simulink model "multirotor_simulation"  (R2025b)
settings: Solver=ode4  StartTime=0.0  StopTime=21  FixedStep=ST  RelTol=1e-3
values from neighbouring files (symbols this model uses):
  a0 = 0    [multirotor_start.m]
  ASLOPE = 5.9    [multirotor_start.m]
  Ax = 0.023    [multirotor_start.m]
  Ay = 0.023    [multirotor_start.m]
  Az = 0.106    [multirotor_start.m]
  BLADES = 2    [multirotor_start.m]
  BLCG = 0    [multirotor_start.m]
  BLCP = 0    [multirotor_start.m]
  BLH1 = b*sind(30)    [multirotor_start.m]
  BLH2 = b    (= 0.275)    [multirotor_start.m]
  BLH3 = b*sind(30)    [multirotor_start.m]
  BLH4 = -b*sind(30)    [multirotor_start.m]
  BLH5 = -b    (= -0.275)    [multirotor_start.m]
  BLH6 = -b*sind(30)    [multirotor_start.m]
  chi1 = 1    [multirotor_start.m]
  chi2 = -1    [multirotor_start.m]
  chi3 = 1    [multirotor_start.m]
  chi4 = -1    [multirotor_start.m]
  chi5 = 1    [multirotor_start.m]
  chi6 = -1    [multirotor_start.m]
  CHORD = 17.55e-3    (= 0.01755)    [multirotor_start.m]
  CHORD75 = 21e-3    (= 0.021)    [multirotor_start.m]
  controller_mode = 1    [multirotor_start.m]
  del_sp = [0 0.7 0 0]'    [multirotor_start.m]
  dyn_visco = 17.89e-6    (= 1.789e-05)    [multirotor_start.m]
  g0 = 9.80665    [multirotor_start.m]
  href = 0    [multirotor_start.m]
  k_ind = 1.35    [multirotor_start.m]
  k_Omega = 14.92    [multirotor_start.m]
  latref = 44.200626    [multirotor_start.m]
  lonref = 12.063822    [multirotor_start.m]
  m = 2.15    [multirotor_start.m]
  MC_ATT_PITCH = 30*pi/180    (= 0.523598775598)    [multirotor_start.m]
  MC_ATT_ROLL = 30*pi/180    (= 0.523598775598)    [multirotor_start.m]
  MC_ATT_YAW = 180*pi/180    (= 3.14159265359)    [multirotor_start.m]
  MC_PITCH_P = 3    [multirotor_start.m]
  MC_PITCHRATE_D = 0    [multirotor_start.m]
  MC_PITCHRATE_I = 0.1*0.5    (= 0.05)    [multirotor_start.m]
  MC_PITCHRATE_P = 0.09    [multirotor_start.m]
  MC_ROLL_P = 3    [multirotor_start.m]
  MC_ROLLRATE_D = 0    [multirotor_start.m]
  MC_ROLLRATE_I = 0.1*0.5    (= 0.05)    [multirotor_start.m]
  MC_ROLLRATE_P = 0.09    [multirotor_start.m]
  MC_VEL_FWD = 5    [multirotor_start.m]
  MC_VEL_FWD_OPT = 0.5    [multirotor_start.m]
  MC_VEL_LAT = 5    [multirotor_start.m]
  MC_VEL_LAT_OPT = 0.5    [multirotor_start.m]
  MC_VEL_VERT = 1    [multirotor_start.m]
  MC_YAW_P = 1.8*0.5    (= 0.9)    [multirotor_start.m]
  MC_YAWRATE_D = 0    [multirotor_start.m]
  MC_YAWRATE_I = 0.1*0    (= 0)    [multirotor_start.m]
  MC_YAWRATE_P = 0.175*0.4    (= 0.07)    [multirotor_start.m]
  MPC_XY_VEL_D_ACC = 0.2*2    (= 0.4)    [multirotor_start.m]
  MPC_XY_VEL_I_ACC = 0.8    [multirotor_start.m]
  MPC_XY_VEL_P_ACC = 1.7*3/3    (= 1.7)    [multirotor_start.m]
  MPC_Z_VEL_D_ACC = 0    [multirotor_start.m]
  MPC_Z_VEL_I_ACC = 2    [multirotor_start.m]
  MPC_Z_VEL_P_ACC = 4    [multirotor_start.m]
  n = 0.6359    [multirotor_start.m]
  p00 = 7.145e-2    (= 0.07145)    [multirotor_start.m]
  p01 = 0.4377    [multirotor_start.m]
  p02 = -10.13    [multirotor_start.m]
  p10 = 1.259e-3    (= 0.001259)    [multirotor_start.m]
  p11 = 1.284e-3    (= 0.001284)    [multirotor_start.m]
  p20 = -7.513e-7    (= -7.513e-07)    [multirotor_start.m]
  PWM_hover = (PWM_idle+PWM_max)/2    (= 1550)    [multirotor_start.m]
  PWM_idle = 1100    [multirotor_start.m]
  PWM_max = 2000    [multirotor_start.m]
  ROTOR = 4*0.0254    (= 0.1016)    [multirotor_start.m]
  set_point_input = 0    [multirotor_start.m]
  ST = 0.01    [multirotor_start.m]
  STACG = 0    [multirotor_start.m]
  STACP = 0    [multirotor_start.m]
  STAH1 = -b*cosd(30)    [multirotor_start.m]
  STAH2 = 0    [multirotor_start.m]
  STAH3 = b*cosd(30)    [multirotor_start.m]
  STAH4 = b*cosd(30)    [multirotor_start.m]
  STAH5 = 0    [multirotor_start.m]
  STAH6 = -b*cosd(30)    [multirotor_start.m]
  TERMINAL_SPEED = 0.5    [multirotor_start.m]
  Theta0 = 45*pi/180    (= 0.785398163397)    [multirotor_start.m]
  THETT = -38.0973*pi/180    (= -0.66492332112)    [multirotor_start.m]
  V_sin_x = 0.3    [multirotor_start.m]
  Vsp = [0 1 0]'    [multirotor_start.m]
  wind_rate = [0 0 0]'    [multirotor_start.m]
  wind_velocity_e = [0 0 0]'    [multirotor_start.m]
  WLCG = -0.03    [multirotor_start.m]
  WLCP = -0.08    [multirotor_start.m]
  WLH1 = 32e-3    (= 0.032)    [multirotor_start.m]
  WLH2 = 32e-3    (= 0.032)    [multirotor_start.m]
  WLH3 = 32e-3    (= 0.032)    [multirotor_start.m]
  WLH4 = 32e-3    (= 0.032)    [multirotor_start.m]
  WLH5 = 32e-3    (= 0.032)    [multirotor_start.m]
  WLH6 = 32e-3    (= 0.032)    [multirotor_start.m]
  Xe_target = Xe_0 + [2, 3, -10]'    [multirotor_start.m]
undefined symbols (not defined in the file or in its folder): fspecial, gray, Rec, SDTV, Sim3dSensor, X, Y, Z
libraries: sm_lib x258, slpidlib x18, nesl_utility x15, sharedtransform x4, simulink x3, aerolibanimutils x2, sim3dcameralib x2, dspvision x2, uavsim3dlib x2, aerolibutil x2, visionconversions x1, visionanalysis x1
(part 1 of 10)
settings Model: Creator=pries  LastModifiedBy=pries
settings RTWCC: GPUComputeCapability=3.5

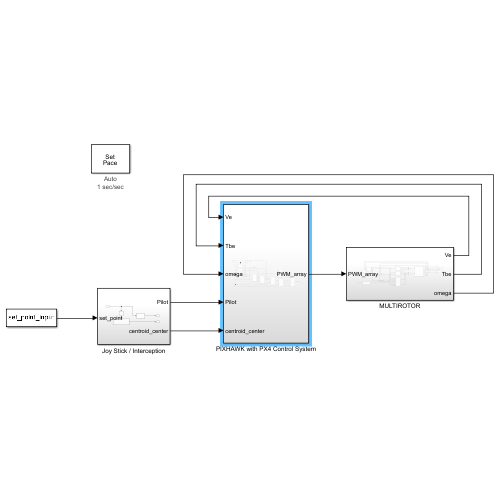
[thumbnail: Simulink's stored preview of the top-level diagram]
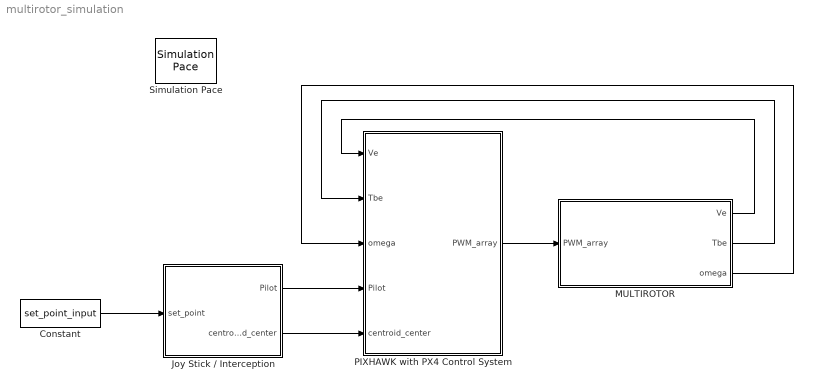
== system multirotor_simulation ==
  Constant : Constant  Value=set_point_input
  Joy Stick / Interception : Subsystem
  MULTIROTOR : Subsystem
  PIXHAWK with PX4 Control System : Subsystem
  Simulation Pace : aerolibanimutils/Simulation Pace  SimulationPace=1  SleepMode=Auto  OutputPaceError=off  SampleTime=ST
  wires:
  PIXHAWK with PX4 Control System/1(PWM_array) -> MULTIROTOR/1(PWM_array)
  MULTIROTOR/1(Ve) -> PIXHAWK with PX4 Control System/1(Ve)
  MULTIROTOR/2(Tbe) -> PIXHAWK with PX4 Control System/2(Tbe)
  MULTIROTOR/3(omega) -> PIXHAWK with PX4 Control System/3(omega)
  Constant/1 -> Joy Stick / Interception/1(set_point)
  Joy Stick / Interception/1(Pilot) -> PIXHAWK with PX4 Control System/4(Pilot)
  Joy Stick / Interception/2(centroid_center) -> PIXHAWK with PX4 Control System/5(centroid_center)

== system multirotor_simulation/Joy Stick // Interception ==
  set_point : Inport
  Compare To Constant : simulink/Logic and Bit Operations/Compare To Constant  relop===  const=0  OutDataTypeStr=boolean
  GCS : Subsystem
  HUSKYLENS : Subsystem
  Pilot : Outport
  centroid_center : Outport  Port=2
  wires:
  HUSKYLENS/1(centroid_center) -> centroid_center/1
  Compare To Constant/1 -> HUSKYLENS/Enable
  GCS/1(Pilot) -> Pilot/1
  set_point/1 -> Compare To Constant/1, GCS/1(set_point)

== system multirotor_simulation/MULTIROTOR ==
  PWM_array : Inport
  3D : Subsystem
  6DOF (Euler Angles) : aerolibobsolete/6DOF (Euler Angles)  units=Metric (MKS)  mtype=Fixed  rep=Euler Angles  xme_0=Xe_0  Vm_0=V0  eul_0=euler0  pm_0=omega0  mass_0=m  mass_e=0.5  mass_f=2.0  inertia=J  inertia_e=eye(3)  inertia_f=2*eye(3)  k_quat=1.0  vre_flag=on  abi_flag=off  aMode=0  xme_statename=''  Vm_statename=''  eul_statename=''  quat_statename=''  pm_statename=''  mass_statename=''
  Add : Sum  Inputs=+++
  Add1 : Sum  Inputs=+++
  Add2 : Sum  Inputs=+-
  Add3 : Sum  Inputs=+-
  Constant : Constant
  ENVIRONMENT : Subsystem
  ESC + MOTOR : Subsystem
  FRAME : Subsystem
  GRAVITY : Subsystem
  MULTIPLE ROTORS FORCES AND MOMENTS : Subsystem
  Terminator1 : Terminator
  Terminator2 : Terminator
  Ve : Outport
  Tbe : Outport  Port=2
  omega : Outport  Port=3
  wires:
  ENVIRONMENT/2(g) -> MULTIPLE ROTORS FORCES AND MOMENTS/6(g), GRAVITY/1(g)
  ENVIRONMENT/1(rho) -> MULTIPLE ROTORS FORCES AND MOMENTS/1(rho), FRAME/1(rho)
  FRAME/2(M_frame) -> Add1/3
  ENVIRONMENT/4(wind_rate) -> Add3/2
  GRAVITY/1(F_grav) -> Add/1
  GRAVITY/2(M_grav) -> Add1/2
  Add/1 -> 6DOF (Euler Angles)/1
  FRAME/1(F_frame) -> Add/2
  6DOF (Euler Angles)/4 -> Tbe/1, ENVIRONMENT/2(Tbe)  "rotation from earth to body frame => Attitude Matrix"
  MULTIPLE ROTORS FORCES AND MOMENTS/2(M_rotor) -> Add1/1
  Add2/1 -> MULTIPLE ROTORS FORCES AND MOMENTS/2(TAS), FRAME/2(TAS)  "TAS"
  6DOF (Euler Angles)/2 -> 3D/1(NED position [m]), ENVIRONMENT/1(Xe)  "position"
  Add3/1 -> MULTIPLE ROTORS FORCES AND MOMENTS/3(omega_TAS)  "omega_TAS"
  6DOF (Euler Angles)/6 -> omega/1, Add3/1, MULTIPLE ROTORS FORCES AND MOMENTS/4(omega)
  Add1/1 -> 6DOF (Euler Angles)/2
  ENVIRONMENT/3(wind_velocity) -> Add2/2  "wind velocity in body frame"
  MULTIPLE ROTORS FORCES AND MOMENTS/1(F_rotor) -> Add/3
  Constant/1 -> MULTIPLE ROTORS FORCES AND MOMENTS/7(h)
  PWM_array/1 -> ESC + MOTOR/1(PWM_array)
  ESC + MOTOR/1(Omega_array) -> MULTIPLE ROTORS FORCES AND MOMENTS/5(Omega_array)
  6DOF (Euler Angles)/3 -> 3D/2(euler_angles [rad])
  6DOF (Euler Angles)/7 -> Terminator1/1
  6DOF (Euler Angles)/8 -> Terminator2/1
  6DOF (Euler Angles)/1 -> Ve/1
  6DOF (Euler Angles)/5 -> Add2/1  "velocity in body frame"

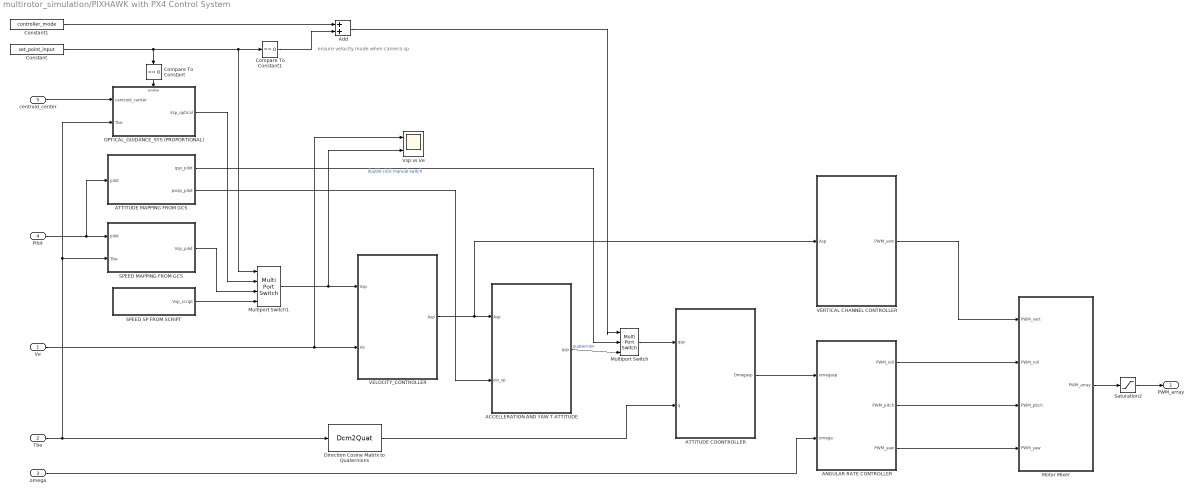
== system multirotor_simulation/PIXHAWK with PX4 Control System ==
  note: ensure velocity mode when camera sp
  Ve : Inport
  Tbe : Inport  Port=2
  omega : Inport  Port=3
  Pilot : Inport  Port=4
  centroid_center : Inport  Port=5
  ACCELLERATION AND YAW T ATTITUDE : Subsystem
  ANGULAR RATE CONTROLLER : Subsystem
  ATTITUDE COONTROLLER : Subsystem
  ATTITUDE MAPPING FROM GCS : Subsystem
  Add : Sum
  Compare To Constant : simulink/Logic and Bit Operations/Compare To Constant  relop===  const=0  OutDataTypeStr=boolean
  Compare To Constant1 : simulink/Logic and Bit Operations/Compare To Constant  relop===  const=0  OutDataTypeStr=boolean
  Constant : Constant  Value=set_point_input
  Constant1 : Constant  Value=controller_mode
  Direction Cosine Matrix to Quaternions : Dcm2Quat
  Motor Mixer : MATLAB Function  TreatAsAtomicUnit=on
  Multiport Switch : MultiPortSwitch  DataPortOrder=Zero-based contiguous  Inputs=2  DiagnosticForDefault=None  zeroidx=on  SaturateOnIntegerOverflow=off  InputSameDT=off
  Multiport Switch1 : MultiPortSwitch  DataPortOrder=Zero-based contiguous  DiagnosticForDefault=None  zeroidx=on  SaturateOnIntegerOverflow=off  InputSameDT=off
  OPTICAL_GUIDANCE_SYS (PROPORTIONAL) : Subsystem
  SPEED MAPPING FROM GCS : Subsystem
  SPEED SP FROM SCRIPT : Subsystem
  Saturation2 : Saturate  UpperLimit=PWM_max  LowerLimit=PWM_idle+10
  VELOCITY_CONTROLLER : Subsystem
  VERTICAL CHANNEL CONTROLLER : Subsystem
  Vsp vs Ve : Scope  NumInputPorts=2
      settings: ActiveDisplayYMinimum=-0.60759896958652782  ActiveDisplayYMaximum=0.44361434408716943
  PWM_array : Outport
  wires:
  VELOCITY_CONTROLLER/1(Asp) -> ACCELLERATION AND YAW T ATTITUDE/1(Asp), VERTICAL CHANNEL CONTROLLER/1(Asp)
  ANGULAR RATE CONTROLLER/3(PWM_yaw) -> Motor Mixer/4(PWM_yaw)
  omega/1 -> ANGULAR RATE CONTROLLER/2(omega)
  Tbe/1 -> Direction Cosine Matrix to Quaternions/1, OPTICAL_GUIDANCE_SYS (PROPORTIONAL)/2(Tbe), SPEED MAPPING FROM GCS/2(Tbe)
  Direction Cosine Matrix to Quaternions/1 -> ATTITUDE COONTROLLER/2(q)
  Ve/1 -> Vsp vs Ve/1, VELOCITY_CONTROLLER/2(Ve)
  ANGULAR RATE CONTROLLER/1(PWM_roll) -> Motor Mixer/2(PWM_roll)
  ANGULAR RATE CONTROLLER/2(PWM_pitch) -> Motor Mixer/3(PWM_pitch)
  Motor Mixer/1(PWM_array) -> Saturation2/1
  VERTICAL CHANNEL CONTROLLER/1(PWM_vert) -> Motor Mixer/1(PWM_vert)
  ATTITUDE COONTROLLER/1(Omegasp) -> ANGULAR RATE CONTROLLER/1(omegasp)
  Pilot/1 -> ATTITUDE MAPPING FROM GCS/1(pilot), SPEED MAPPING FROM GCS/1(pilot)
  ATTITUDE MAPPING FROM GCS/2(psisp_pilot) -> ACCELLERATION AND YAW T ATTITUDE/2(psi_sp)
  ACCELLERATION AND YAW T ATTITUDE/1(qsp) -> Multiport Switch/3  "quaternion"
  Multiport Switch/1 -> ATTITUDE COONTROLLER/1(qsp)
  ATTITUDE MAPPING FROM GCS/1(qsp_pilot) -> Multiport Switch/2  "double click manual switch"
  centroid_center/1 -> OPTICAL_GUIDANCE_SYS (PROPORTIONAL)/1(centroid_center)
  Saturation2/1 -> PWM_array/1
  Multiport Switch1/1 -> Vsp vs Ve/2, VELOCITY_CONTROLLER/1(Vsp)
  Constant/1 -> Compare To Constant1/1, Multiport Switch1/1, Compare To Constant/1
  Compare To Constant/1 -> OPTICAL_GUIDANCE_SYS (PROPORTIONAL)/Enable
  SPEED MAPPING FROM GCS/1(Vsp_pilot) -> Multiport Switch1/3
  OPTICAL_GUIDANCE_SYS (PROPORTIONAL)/1(Vsp_optical) -> Multiport Switch1/2
  Constant1/1 -> Add/1
  Compare To Constant1/1 -> Add/2
  Add/1 -> Multiport Switch/1
  SPEED SP FROM SCRIPT/1(Vsp_script) -> Multiport Switch1/4

== system multirotor_simulation/Joy Stick // Interception/GCS ==
  set_point : Inport
  1-D Lookup Table : Lookup_n-D  NumberOfTableDimensions=1  BreakpointsForDimension1=[0 1]  Table=[-1 1]  InternalRulePriority=Speed  RndMeth=Simplest
  Constant1 : Constant  Value=del_sp
  Demux : Demux  Outputs=6
  Multiport Switch : MultiPortSwitch  Inputs=2  DiagnosticForDefault=None  SaturateOnIntegerOverflow=off  InputSameDT=off
  Mux : Mux
  Pilot Joystick All : aerolibanimutils/Pilot Joystick  JoystickID=None  OutputConfiguration=AllOutputs  SampleTime=ST
      settings: LibrarySourceBlock=aerolibanimutils/Pilot Joystick All
  Terminator{,1..3} (4 alike) : Terminator
  Pilot : Outport
  wires:
  1-D Lookup Table/1 -> Mux/1  "thrust [-1,1]"
  Demux/6 -> Terminator3/1
  Demux/5 -> Terminator2/1
  Demux/2 -> Mux/3  "pitch [-1,1]"
  Demux/4 -> Mux/4  "yaw [-1,1]"
  Demux/1 -> Mux/2  "roll [-1,1]"
  Pilot Joystick All/2 -> Terminator1/1
  Demux/3 -> 1-D Lookup Table/1
  Pilot Joystick All/1 -> Demux/1
  Pilot Joystick All/3 -> Terminator/1
  set_point/1 -> Multiport Switch/1
  Mux/1 -> Multiport Switch/2
  Constant1/1 -> Multiport Switch/3
  Multiport Switch/1 -> Pilot/1

== system multirotor_simulation/Joy Stick // Interception/HUSKYLENS ==
  Enable : EnablePort
  OPTICAL_SENSOR : Subsystem
  VISION_DETECTION_SOFTWARE : Subsystem
  centroid_center : Outport
  wires:
  OPTICAL_SENSOR/1(Image) -> VISION_DETECTION_SOFTWARE/1(Image)
  VISION_DETECTION_SOFTWARE/1(centroid_center) -> centroid_center/1

== system multirotor_simulation/MULTIROTOR/3D ==
  NED position [m] : Inport
  euler_angles [rad] : Inport  Port=2
  SIMECHANICS 3D SCENE : Subsystem  Commented=on
  UNREAL ENGINE 3D SCENE : Subsystem
  wires:
  NED position [m]/1 -> UNREAL ENGINE 3D SCENE/1(NED position [m]), SIMECHANICS 3D SCENE/1(NED position [m])
  euler_angles [rad]/1 -> UNREAL ENGINE 3D SCENE/2(euler_angles [rad]), SIMECHANICS 3D SCENE/2(euler_angles [rad])

== system multirotor_simulation/MULTIROTOR/ENVIRONMENT ==
  Xe : Inport
  Tbe : Inport  Port=2
  Constant : Constant  Value=href
  Constant1 : Constant  Value=wind_velocity_e
  Constant2 : Constant  Value=wind_rate
  Flat Earth to LLA : FlatEarth2LLA  R=6378137  LL0=[latref lonref]
  ISA Atmosphere Model : aerolibatmos2/ISA Atmosphere Model  useExtended=off  action=None  custom=off  viscosityOut=off  g=9.80665  gamma=1.4  R=287.0531  L=0.0065  h_trop=11000  h_strat=20000  rho0=1.225  P0=101325  T0=288.15  h0=0  S=110.4  Tref=273.15  muref=1.716e-5
  Matrix Multiply : Product  Multiplication=Matrix(*)
  Matrix Multiply1 : Product  Multiplication=Matrix(*)
  Mux : Mux  Inputs=[2 1]
  Reshape transforms inp to req out : Reshape
  Terminator : Terminator
  Terminator1 : Terminator
  Terminator2 : Terminator
  "WGS84 Gravity Model  " : GravityWGS84
  rho : Outport
  g : Outport  Port=2
  wind_velocity : Outport  Port=3
  wind_rate : Outport  Port=4
  wires:
  ISA Atmosphere Model/1 -> Terminator/1
  Mux/1 -> Reshape transforms inp to req out/1
  ISA Atmosphere Model/3 -> Terminator2/1
  "WGS84 Gravity Model  "/1 -> Matrix Multiply/2
  Flat Earth to LLA/2 -> ISA Atmosphere Model/1, Mux/2
  Constant/1 -> Flat Earth to LLA/2
  ISA Atmosphere Model/2 -> Terminator1/1
  Reshape transforms inp to req out/1 -> "WGS84 Gravity Model  "/1
  Flat Earth to LLA/1 -> Mux/1
  ISA Atmosphere Model/4 -> rho/1
  Matrix Multiply/1 -> g/1
  Xe/1 -> Flat Earth to LLA/1
  Constant2/1 -> wind_rate/1
  Tbe/1 -> Matrix Multiply1/1, Matrix Multiply/1
  Matrix Multiply1/1 -> wind_velocity/1
  Constant1/1 -> Matrix Multiply1/2

== system multirotor_simulation/MULTIROTOR/ESC + MOTOR ==
  PWM_array : Inport
  Constant : Constant  Value=k_Omega
  Constant1 : Constant  Value=n
  Constant2 : Constant  Value=PWM_idle
  DJI OPTO 30A + DJI 2212 : MATLAB Function  TreatAsAtomicUnit=on
  Omega_array : Outport
  wires:
  Constant1/1 -> DJI OPTO 30A + DJI 2212/2(n)
  Constant2/1 -> DJI OPTO 30A + DJI 2212/3(PWM_idle)
  DJI OPTO 30A + DJI 2212/1(Omega_array) -> Omega_array/1
  Constant/1 -> DJI OPTO 30A + DJI 2212/1(k_Omega)
  PWM_array/1 -> DJI OPTO 30A + DJI 2212/4(PWM_array)

== system multirotor_simulation/MULTIROTOR/FRAME ==
  rho : Inport
  TAS : Inport  Port=2
  Constant1 : Constant  Value=Ay
  Constant10 : Constant  Value=WLCP
  Constant11 : Constant  Value=Ax
  Constant2 : Constant  Value=Az
  Constant3 : Constant  Value=STACP
  Constant6 : Constant  Value=BLCP
  Constant7 : Constant  Value=WLCP
  Constant8 : Constant  Value=STACG
  Constant9 : Constant  Value=BLCG
  MATLAB Function : MATLAB Function  TreatAsAtomicUnit=on
  F_frame : Outport
  M_frame : Outport  Port=2
  wires:
  MATLAB Function/1(F_frame) -> F_frame/1
  Constant3/1 -> MATLAB Function/4(STACP)
  Constant10/1 -> MATLAB Function/9(WLCG)
  Constant9/1 -> MATLAB Function/8(BLCG)
  TAS/1 -> MATLAB Function/11(TAS)
  Constant1/1 -> MATLAB Function/2(Ay)
  Constant6/1 -> MATLAB Function/5(BLCP)
  Constant2/1 -> MATLAB Function/3(Az)
  Constant11/1 -> MATLAB Function/1(Ax)
  Constant8/1 -> MATLAB Function/7(STACG)
  Constant7/1 -> MATLAB Function/6(WLCP)
  rho/1 -> MATLAB Function/10(rho)
  MATLAB Function/2(M_frame) -> M_frame/1

== system multirotor_simulation/MULTIROTOR/GRAVITY ==
  g : Inport
  Constant : Constant  Value=0
  Gain : Gain  Gain=m
  F_grav : Outport
  M_grav : Outport  Port=2
  wires:
  Gain/1 -> F_grav/1
  Constant/1 -> M_grav/1
  g/1 -> Gain/1

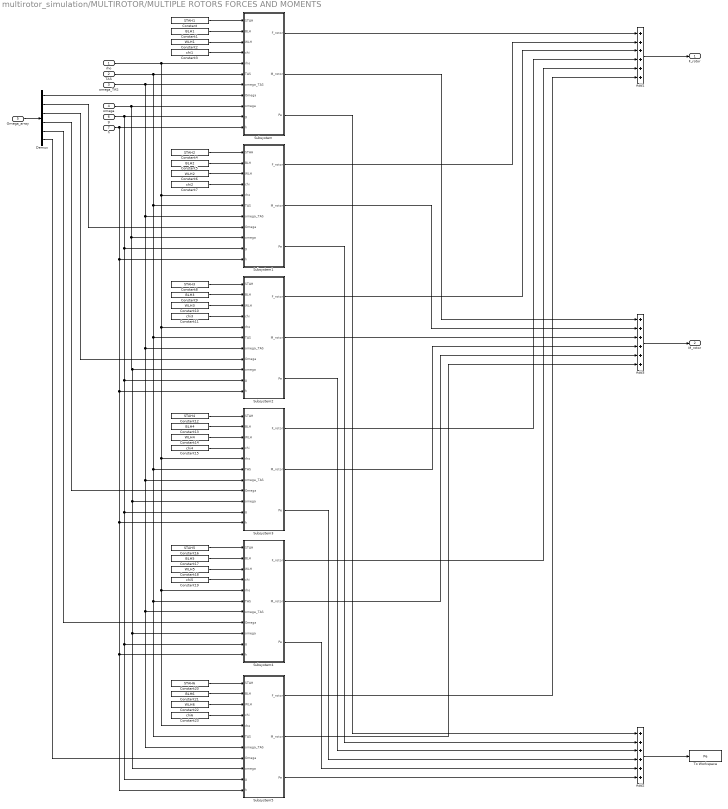
== system multirotor_simulation/MULTIROTOR/MULTIPLE ROTORS FORCES AND MOMENTS ==
  rho : Inport
  TAS : Inport  Port=2
  omega_TAS : Inport  Port=3
  omega : Inport  Port=4
  Omega_array : Inport  Port=5
  g : Inport  Port=6
  h : Inport  Port=7
  Add1 : Sum  Inputs=++++++
  Add2 : Sum  Inputs=++++++
  Add3 : Sum  Inputs=++++++
  Constant : Constant  Value=STAH1
  Constant1 : Constant  Value=BLH1
  Constant10 : Constant  Value=WLH3
  Constant11 : Constant  Value=chi3
  Constant12 : Constant  Value=STAH4
  Constant13 : Constant  Value=BLH4
  Constant14 : Constant  Value=WLH4
  Constant15 : Constant  Value=chi4
  Constant16 : Constant  Value=STAH5
  Constant17 : Constant  Value=BLH5
  Constant18 : Constant  Value=WLH5
  Constant19 : Constant  Value=chi5
  Constant2 : Constant  Value=WLH1
  Constant20 : Constant  Value=STAH6
  Constant21 : Constant  Value=BLH6
  Constant22 : Constant  Value=WLH6
  Constant23 : Constant  Value=chi6
  Constant3 : Constant  Value=chi1
  Constant4 : Constant  Value=STAH2
  Constant5 : Constant  Value=BLH2
  Constant6 : Constant  Value=WLH2
  Constant7 : Constant  Value=chi2
  Constant8 : Constant  Value=STAH3
  Constant9 : Constant  Value=BLH3
  Demux : Demux  Outputs=6
  Subsystem : Subsystem
  Subsystem1 : Subsystem
  Subsystem2 : Subsystem
  Subsystem3 : Subsystem
  Subsystem4 : Subsystem
  Subsystem5 : Subsystem
  To Workspace : ToWorkspace  VariableName=Pe  SampleTime=-1
  F_rotor : Outport
  M_rotor : Outport  Port=2
  wires:
  Constant/1 -> Subsystem/1(STAH)
  Constant21/1 -> Subsystem5/2(BLH)
  Add3/1 -> M_rotor/1
  Constant17/1 -> Subsystem4/2(BLH)
  Constant7/1 -> Subsystem1/4(chi)
  Subsystem2/2(M_rotor) -> Add3/3
  Subsystem4/3(Pe) -> Add2/5
  h/1 -> Subsystem5/11(h), Subsystem4/11(h), Subsystem3/11(h), Subsystem2/11(h), Subsystem1/11(h), Subsystem/11(h)
  Constant5/1 -> Subsystem1/2(BLH)
  Constant8/1 -> Subsystem2/1(STAH)
  Constant3/1 -> Subsystem/4(chi)
  Subsystem2/3(Pe) -> Add2/3
  Constant12/1 -> Subsystem3/1(STAH)
  Subsystem4/2(M_rotor) -> Add3/5
  Subsystem/2(M_rotor) -> Add3/1
  Constant16/1 -> Subsystem4/1(STAH)
  Constant19/1 -> Subsystem4/4(chi)
  Constant6/1 -> Subsystem1/3(WLH)
  Constant13/1 -> Subsystem3/2(BLH)
  Constant20/1 -> Subsystem5/1(STAH)
  omega/1 -> Subsystem/9(omega), Subsystem1/9(omega), Subsystem5/9(omega), Subsystem4/9(omega), Subsystem3/9(omega), Subsystem2/9(omega)
  Constant2/1 -> Subsystem/3(WLH)
  Subsystem2/1(F_rotor) -> Add1/3
  Constant15/1 -> Subsystem3/4(chi)
  Subsystem5/1(F_rotor) -> Add1/6
  Constant10/1 -> Subsystem2/3(WLH)
  Subsystem3/3(Pe) -> Add2/4
  Subsystem3/1(F_rotor) -> Add1/4
  Constant18/1 -> Subsystem4/3(WLH)
  Constant1/1 -> Subsystem/2(BLH)
  g/1 -> Subsystem/10(g), Subsystem5/10(g), Subsystem4/10(g), Subsystem3/10(g), Subsystem2/10(g), Subsystem1/10(g)
  rho/1 -> Subsystem5/5(rho), Subsystem4/5(rho), Subsystem3/5(rho), Subsystem2/5(rho), Subsystem1/5(rho), Subsystem/5(rho)
  Add1/1 -> F_rotor/1
  Subsystem1/3(Pe) -> Add2/2
  Subsystem/3(Pe) -> Add2/1
  Subsystem3/2(M_rotor) -> Add3/4
  Add2/1 -> To Workspace/1
  TAS/1 -> Subsystem5/6(TAS), Subsystem4/6(TAS), Subsystem3/6(TAS), Subsystem2/6(TAS), Subsystem1/6(TAS), Subsystem/6(TAS)
  Constant22/1 -> Subsystem5/3(WLH)
  Constant9/1 -> Subsystem2/2(BLH)
  Constant23/1 -> Subsystem5/4(chi)
  Constant14/1 -> Subsystem3/3(WLH)
  Constant11/1 -> Subsystem2/4(chi)
  Constant4/1 -> Subsystem1/1(STAH)
  Subsystem5/2(M_rotor) -> Add3/6
  Subsystem1/1(F_rotor) -> Add1/2
  Subsystem/1(F_rotor) -> Add1/1
  omega_TAS/1 -> Subsystem5/7(omega_TAS), Subsystem4/7(omega_TAS), Subsystem3/7(omega_TAS), Subsystem2/7(omega_TAS), Subsystem1/7(omega_TAS), Subsystem/7(omega_TAS)
  Subsystem4/1(F_rotor) -> Add1/5
  Subsystem5/3(Pe) -> Add2/6
  Omega_array/1 -> Demux/1
  Demux/2 -> Subsystem1/8(Omega)
  Demux/3 -> Subsystem2/8(Omega)
  Demux/4 -> Subsystem3/8(Omega)
  Demux/5 -> Subsystem4/8(Omega)
  Demux/6 -> Subsystem5/8(Omega)
  Demux/1 -> Subsystem/8(Omega)
  Subsystem1/2(M_rotor) -> Add3/2

== system multirotor_simulation/PIXHAWK with PX4 Control System/ACCELLERATION AND YAW T ATTITUDE ==
  Asp : Inport
  psi_sp : Inport  Port=2
  Constant : Constant  Value=g0
  MATLAB Function : MATLAB Function  TreatAsAtomicUnit=on
  Mux : Mux  Inputs=3
  Rotation Angles to Quaternions : sharedtransform/Rotation Angles to Quaternions  rotationOrder=ZYX  aMode=aMode
  qsp : Outport
  wires:
  Constant/1 -> MATLAB Function/2(g0)
  psi_sp/1 -> Mux/1, MATLAB Function/3(psi_sp)
  Asp/1 -> MATLAB Function/1(Asp)
  MATLAB Function/2(phi_sp) -> Mux/3
  MATLAB Function/1(theta_sp) -> Mux/2
  Mux/1 -> Rotation Angles to Quaternions/1
  Rotation Angles to Quaternions/1 -> qsp/1

== system multirotor_simulation/PIXHAWK with PX4 Control System/ANGULAR RATE CONTROLLER ==
  omegasp : Inport
  omega : Inport  Port=2
  Gain : Gain  Gain=0.5*(PWM_max-PWM_idle)
  Gain1 : Gain  Gain=0.5*(PWM_max-PWM_idle)
  Gain2 : Gain  Gain=0.5*(PWM_max-PWM_idle)
  PITCH_RATE_CONTROLLER : Subsystem
  ROLL_RATE_CONTROLLER : Subsystem
  YAW_RATE_CONTROLLER : Subsystem
  PWM_roll : Outport
  PWM_pitch : Outport  Port=2
  PWM_yaw : Outport  Port=3
  wires:
  omegasp/1 -> ROLL_RATE_CONTROLLER/1(omegasp), PITCH_RATE_CONTROLLER/1(omegasp), YAW_RATE_CONTROLLER/1(omegasp)
  omega/1 -> YAW_RATE_CONTROLLER/2(omega), PITCH_RATE_CONTROLLER/2(omega), ROLL_RATE_CONTROLLER/2(omega)
  YAW_RATE_CONTROLLER/1(delta_yaw) -> Gain2/1
  PITCH_RATE_CONTROLLER/1(delta_pitchl) -> Gain1/1
  ROLL_RATE_CONTROLLER/1(delta_roll) -> Gain/1
  Gain/1 -> PWM_roll/1
  Gain1/1 -> PWM_pitch/1
  Gain2/1 -> PWM_yaw/1

== system multirotor_simulation/PIXHAWK with PX4 Control System/ATTITUDE COONTROLLER ==
  qsp : Inport
  q : Inport  Port=2
  Constant : Constant  Value=MC_ROLL_P
  Constant1 : Constant  Value=MC_PITCH_P
  Constant2 : Constant  Value=MC_YAW_P
  MATLAB Function : MATLAB Function  TreatAsAtomicUnit=on
  Quaternion Conjugate : aerolibutil/Quaternion Conjugate
  Quaternion Multiplication : aerolibutil/Quaternion Multiplication
  Quaternion Normalize : sharedutil/Quaternion Normalize  aMode=aMode
  Omegasp : Outport
  wires:
  Constant2/1 -> MATLAB Function/4(MC_YAW_P)
  Constant1/1 -> MATLAB Function/3(MC_PITCH_P)
  qsp/1 -> Quaternion Multiplication/2
  Constant/1 -> MATLAB Function/2(MC_ROLL_P)
  Quaternion Normalize/1 -> Quaternion Multiplication/1  "should already be normal => eliminate numerical noise"
  Quaternion Conjugate/1 -> Quaternion Normalize/1
  Quaternion Multiplication/1 -> MATLAB Function/1(qe)  "qe"
  MATLAB Function/1(Omegasp) -> Omegasp/1
  q/1 -> Quaternion Conjugate/1

== system multirotor_simulation/PIXHAWK with PX4 Control System/ATTITUDE MAPPING FROM GCS ==
  pilot : Inport
  Constant2 : Constant  Value=MC_ATT_ROLL
  Constant3 : Constant  Value=MC_ATT_PITCH
  Constant4 : Constant  Value=MC_ATT_YAW
  MATLAB Function1 : MATLAB Function  TreatAsAtomicUnit=on
  Rotation Angles to Quaternions : sharedtransform/Rotation Angles to Quaternions  rotationOrder=ZYX  aMode=aMode
  Selector : Selector  InputPortWidth=3  IndexOptions=Index vector (dialog)  Indices=[3 2 1]  OutputSizes=1
  Selector1 : Selector  InputPortWidth=3  IndexOptions=Index vector (dialog)  Indices=[3]  OutputSizes=1
  qsp_pilot : Outport
  psisp_pilot : Outport  Port=2
  wires:
  Constant4/1 -> MATLAB Function1/4(MC_ATT_YAW)
  Constant2/1 -> MATLAB Function1/2(MC_ATT_ROLL)
  pilot/1 -> MATLAB Function1/1(pilot)
  Constant3/1 -> MATLAB Function1/3(MC_ATT_PITCH)
  Rotation Angles to Quaternions/1 -> qsp_pilot/1
  MATLAB Function1/1(eulersp_pilot) -> Selector1/1, Selector/1
  Selector/1 -> Rotation Angles to Quaternions/1
  Selector1/1 -> psisp_pilot/1

== system multirotor_simulation/PIXHAWK with PX4 Control System/OPTICAL_GUIDANCE_SYS (PROPORTIONAL) ==
  centroid_center : Inport
  Tbe : Inport  Port=2
  Enable : EnablePort
  Constant2 : Constant  Value=MC_VEL_FWD_OPT
  Constant3 : Constant  Value=MC_VEL_LAT_OPT
  Constant4 : Constant  Value=TERMINAL_SPEED
  Direction Cosine Matrix to Rotation Angles : sharedtransform/Direction Cosine Matrix to Rotation Angles  rotationOrder=ZYX  aMode=aMode  action=None  tolerance=eps(2)
      settings: LibrarySourceBlock=|
      | aerolibtransform2/Direction Cosine Matrix
      | to Rotation Angles
  MATLAB Function1 : MATLAB Function  TreatAsAtomicUnit=on
  Selector : Selector  InputPortWidth=3  IndexOptions=Index vector (dialog)  Indices=[1]  OutputSizes=1
  Vsp_optical : Outport
  wires:
  Constant2/1 -> MATLAB Function1/3(MC_VEL_FWD)
  Constant4/1 -> MATLAB Function1/5(TERMINAL_SPEED)
  Constant3/1 -> MATLAB Function1/4(MC_VEL_LAT)
  centroid_center/1 -> MATLAB Function1/1(centroid_center)
  MATLAB Function1/1(Vsp_optical) -> Vsp_optical/1
  Direction Cosine Matrix to Rotation Angles/1 -> Selector/1
  Tbe/1 -> Direction Cosine Matrix to Rotation Angles/1
  Selector/1 -> MATLAB Function1/2(psi)

== system multirotor_simulation/PIXHAWK with PX4 Control System/SPEED MAPPING FROM GCS ==
  pilot : Inport
  Tbe : Inport  Port=2
  Constant2 : Constant  Value=MC_VEL_FWD
  Constant3 : Constant  Value=MC_VEL_LAT
  Constant4 : Constant  Value=MC_VEL_VERT
  Direction Cosine Matrix to Rotation Angles : sharedtransform/Direction Cosine Matrix to Rotation Angles  rotationOrder=ZYX  aMode=aMode  action=None  tolerance=eps(2)
      settings: LibrarySourceBlock=|
      | aerolibtransform2/Direction Cosine Matrix
      | to Rotation Angles
  MATLAB Function1 : MATLAB Function  TreatAsAtomicUnit=on
  Selector : Selector  InputPortWidth=3  IndexOptions=Index vector (dialog)  Indices=[1]  OutputSizes=1
  Vsp_pilot : Outport
  wires:
  MATLAB Function1/1(Vsp_pilot) -> Vsp_pilot/1
  Constant3/1 -> MATLAB Function1/4(MC_VEL_LAT)
  pilot/1 -> MATLAB Function1/1(pilot)
  Constant2/1 -> MATLAB Function1/3(MC_VEL_FWD)
  Constant4/1 -> MATLAB Function1/5(MC_VEL_VERT)
  Tbe/1 -> Direction Cosine Matrix to Rotation Angles/1  "not psisp => assume control system is so fast psi = psisp"
  Direction Cosine Matrix to Rotation Angles/1 -> Selector/1
  Selector/1 -> MATLAB Function1/2(psisp)

== system multirotor_simulation/PIXHAWK with PX4 Control System/SPEED SP FROM SCRIPT ==
  Constant1 : Constant  Value=V_sin_x
  Constant4 : Constant  Value=Vsp
  MATLAB Function : MATLAB Function  TreatAsAtomicUnit=on
  Sine Wave : Sin  Amplitude=V_sin_x  SampleTime=0
  Vsp_script : Outport
  wires:
  Constant4/1 -> MATLAB Function/1(v_sp)
  MATLAB Function/1(v_sp_out) -> Vsp_script/1
  Sine Wave/1 -> MATLAB Function/2(sin_x)
  Constant1/1 -> MATLAB Function/3(V_sin_x)

== system multirotor_simulation/PIXHAWK with PX4 Control System/VELOCITY_CONTROLLER ==
  Vsp : Inport
  Ve : Inport  Port=2
  Mux : Mux  Inputs=3
  X_SPEED_CONTROLLER : Subsystem
  Y_SPEED_CONTROLLER : Subsystem
  Z_SPEED_CONTROLLER : Subsystem
  Asp : Outport
  wires:
  X_SPEED_CONTROLLER/1(Asp_x) -> Mux/1
  Ve/1 -> Z_SPEED_CONTROLLER/2(V), Y_SPEED_CONTROLLER/2(V), X_SPEED_CONTROLLER/2(V)
  Z_SPEED_CONTROLLER/1(Asp_z) -> Mux/3
  Y_SPEED_CONTROLLER/1(Asp_y) -> Mux/2
  Mux/1 -> Asp/1
  Vsp/1 -> X_SPEED_CONTROLLER/1(Vsp), Y_SPEED_CONTROLLER/1(Vsp), Z_SPEED_CONTROLLER/1(Vsp)

== system multirotor_simulation/PIXHAWK with PX4 Control System/VERTICAL CHANNEL CONTROLLER ==
  Asp : Inport
  Constant1 : Constant  Value=g0
  Constant2 : Constant  Value=PWM_hover
  Gain : Gain  Gain=0.5*(PWM_max-PWM_idle)
  MATLAB Function : MATLAB Function  TreatAsAtomicUnit=on
  Saturation : Saturate  UpperLimit=1  LowerLimit=-1
  Sum : Sum  Inputs=|++
  PWM_vert : Outport
  wires:
  MATLAB Function/1(delta_vert) -> Saturation/1
  Asp/1 -> MATLAB Function/1(Asp)
  Constant1/1 -> MATLAB Function/2(g0)
  Saturation/1 -> Gain/1
  Constant2/1 -> Sum/2
  Gain/1 -> Sum/1
  Sum/1 -> PWM_vert/1

== system multirotor_simulation/Joy Stick // Interception/HUSKYLENS/OPTICAL_SENSOR ==
  Simulation 3D Fisheye Camera : sim3dcameralib/Simulation 3D Fisheye Camera  Priority=1  sensorTag=Sim3dSensor�  sensorId=1  sensorName=Sim3dSensor1  vehTagList={'Scene Origin';'SimulinkVehicle1';'SimulinkVehicle2'}  vehTag=SimulinkVehicle1  CoordinateSystem=ISO8855  mountLoc=Origin  offsetFlag=on  tmountOffset=[0, 0, 0.1]  extTmount=off  rmountOffset=[0, -90, 0]  extRmount=off  OpticalCenter=[320, 320]  ImageSize=[640, 640]  RadialDistortion=[640, 0, 0, 0]  StretchMatrix=[1, 0; 0, 1]  TransformOutportEnabled=off  SampleTime=0.2  mountPoint=[0 0 0.1]  mountOrientation=[0 -90 0]  aMode=4  ID=1
      settings: LibrarySourceBlock=uavsim3dlib/Simulation 3D Fisheye Camera
  Image : Outport
  wires:
  Simulation 3D Fisheye Camera/1 -> Image/1

== system multirotor_simulation/Joy Stick // Interception/HUSKYLENS/VISION_DETECTION_SOFTWARE ==
  Image : Inport
  Centroid Calculation : MATLAB Function  TreatAsAtomicUnit=on
  Color Space Conversion : visionconversions/Color Space  Conversion  conversion=Obsolete  conversionActive=R'G'B' to intensity  wp_str=D65  rec=Rec. 601 (SDTV)  sys=1125/60/2:1  imagePorts=One multidimensional signal
  Corner Detection : visionanalysis/Corner Detection  method=Harris corner detection (Harris & Stephens)  factor=0.02  filter=fspecial('gaussian', [1 5], 1.5)  thrInten=0.1  thrAngle=157.5  output=Obsolete9b  outputInUse=Corner location  maxNum=10  thrMetric=0.0005  neighborSize=[11 11]  isOutVarDim=off  roundingMode=Floor  overflowMode=off  firstCoeffMode=Specify word length  firstCoeffWordLength=16  firstCoeffFracLength=16  prodOutputMode=Binary point scaling  prodOutputWordLength=32  prodOutputFracLength=0  accumMode=Binary point scaling  accumWordLength=32  accumFracLength=0  memoryMode=Binary point scaling  memoryWordLength=32  memoryFracLength=0
  Data Type Conversion : DataTypeConversion  SaturateOnIntegerOverflow=off  RndMeth=Floor
  Low Pass Filter_x : TransferFcn  Denominator=[1 1]
  Low Pass Filter_y : TransferFcn  Denominator=[1 1]
  Mux : Mux  Inputs=2
  Mux1 : Mux  Inputs=2
  Render Huskylens : Subsystem
  Terminator : Terminator
  centroid_center : Outport
  wires:
  Image/1 -> Render Huskylens/1(Image), Color Space Conversion/1
  Centroid Calculation/4(y_centroid_center) -> Low Pass Filter_y/1
  Centroid Calculation/3(x_centroid_center) -> Low Pass Filter_x/1
  Centroid Calculation/2(y_centroid) -> Mux/2
  Centroid Calculation/1(x_centroid) -> Mux/1
  Mux/1 -> Data Type Conversion/1
  Corner Detection/1 -> Centroid Calculation/1(Loc)
  Low Pass Filter_y/1 -> Mux1/2
  Low Pass Filter_x/1 -> Mux1/1
  Mux1/1 -> centroid_center/1
  Corner Detection/2 -> Terminator/1
  Color Space Conversion/1 -> Corner Detection/1
  Data Type Conversion/1 -> Render Huskylens/2(Pts)

== system multirotor_simulation/MULTIROTOR/3D/SIMECHANICS 3D SCENE ==
  NED position [m] : Inport
  euler_angles [rad] : Inport  Port=2
  Constant{1..2,5..8} (6 alike) : Constant  Value=[0 0 0]'
  Constant3 : Constant  Value=0
  Mux : Mux  Inputs=2
  Selector : Selector  InputPortWidth=3  IndexOptions=Index vector (dialog)  Indices=[1 2]  OutputSizes=1
  SimMechanics : Subsystem
  SimMechanics1 : Subsystem
  Simulink - PS converter : Subsystem
  Simulink - PS converter1 : Subsystem
  wires:
  euler_angles [rad]/1 -> Simulink - PS converter/4(eta)
  NED position [m]/1 -> Selector/1, Simulink - PS converter/2(xi)
  Mux/1 -> Simulink - PS converter1/1(xi)
  Constant5/1 -> Simulink - PS converter/6(dot^2 eta)
  Constant7/1 -> Simulink - PS converter/3(vi)
  Constant8/1 -> Simulink - PS converter/1(ai)
  Constant3/1 -> Mux/2
  Constant2/1 -> Simulink - PS converter1/2(vi)
  Selector/1 -> Mux/1
  Constant1/1 -> Simulink - PS converter1/3(ai)
  Constant6/1 -> Simulink - PS converter/5(dot eta)
  connections:
  Simulink - PS converter/RConn2 -- SimMechanics/LConn2
  Simulink - PS converter/RConn1 -- SimMechanics/LConn1
  Simulink - PS converter/RConn6 -- SimMechanics/LConn6
  Simulink - PS converter/RConn4 -- SimMechanics/LConn4
  Simulink - PS converter/RConn3 -- SimMechanics/LConn3
  Simulink - PS converter1/RConn2 -- SimMechanics1/LConn2
  Simulink - PS converter1/RConn1 -- SimMechanics1/LConn1
  Simulink - PS converter1/RConn3 -- SimMechanics1/LConn3
  Simulink - PS converter/RConn5 -- SimMechanics/LConn5

== system multirotor_simulation/MULTIROTOR/3D/UNREAL ENGINE 3D SCENE ==
  NED position [m] : Inport
  euler_angles [rad] : Inport  Port=2
  Constant1 : Constant  Value=Xe_target
  Constant2 : Constant  Value=[0 0 0]'
  Gain : Gain  Gain=diag([1 -1 -1])  Multiplication=Matrix(K*u) (u vector)
  Gain1 : Gain  Gain=diag([-1 -1 1])  Multiplication=Matrix(K*u) (u vector)
  Gain2 : Gain  Gain=diag([1 -1 -1])  Multiplication=Matrix(K*u) (u vector)
  Gain3 : Gain  Gain=diag([-1 -1 1])  Multiplication=Matrix(K*u) (u vector)
  Selector : Selector  InputPortWidth=3  IndexOptions=Index vector (dialog)  Indices=[3 2 1]  OutputSizes=1
  Selector1 : Selector  InputPortWidth=3  IndexOptions=Index vector (dialog)  Indices=[3 2 1]  OutputSizes=1
  Simulation 3D Camera : sim3dcameralib/Simulation 3D Camera  Priority=1  sensorTag=Sim3dSensor�  sensorId=2  sensorName=Sim3dSensor�  vehTagList={'Scene Origin';'SimulinkVehicle1';'SimulinkVehicle2'}  vehTag=SimulinkVehicle1  CoordinateSystem=ISO8855  mountLoc=Origin  offsetFlag=on  tmountOffset=[-1, -0.7, -2]  extTmount=off  rmountOffset=[0, -70, 0]  extRmount=off  FocalLength=[1109, 1109]  OpticalCenter=[640, 360]  ImageSize=[720, 1280]  RadialDistortion=[0, 0]  TangentialDistortion=[0, 0]  SensorSkew=0  VisualizeFieldOfView=off  FieldOfViewRange=61  DepthOutportEnabled=off  SemanticOutportEnabled=off  TransformOutportEnabled=off  SampleTime=-1  mountPoint=[-1 -0.7 -2]  mountOrientation=[0 -70 0]  aMode=4  ID=2
      settings: LibrarySourceBlock=uavsim3dlib/Simulation 3D Camera
  Simulation 3D Scene Configuration : sim3dlib/Simulation 3D Scene Configuration  Priority=0  ProjectFormat=Default Scenes  SceneDesc=US city block  ProjectName=C:\Program Files\MATLAB\R2025b\toolbox\shared\sim3d_projects\automotive_project_windows\UE\WindowsNoEditor\VehicleSimulation.exe  ScenePath=/Game/Maps/USCityBlock  EnableOpenDRIVE=off  vehTagList={'Custom';'Scene Origin';'SimulinkVehicle1';'SimulinkVehicle2'}  vehTag=SimulinkVehicle1  AttachedCameraRelativeTranslation=[0 0 0]  FreeCameraDefaultInitialTranslation=[-6, 0, 2]  AttachedCameraRelativeRotation=[0 0 0]  FreeCameraDefaultInitialRotation=[0, -15, 0]  ViewpointName=Custom  FreeCameraInitialTranslation=[0 0 0]  ViewpointTranslation=[0 0 0]  FreeCameraInitialRotation=[0 0 0]  ViewpointRotation=[0 0 0]  OpVisEn=off  Ts=0.2  EnableWindow=off  EnableRemoteAccess=off  EnableWeather=off  SunAzimuth=90  SunAltitude=40.0  EnableGeospatialSun=off  Latitude=0  Longitude=0  Date=2023-01-01  Time=10:30:00  GeoTimeZone=-5.0  SunDaylightSaving=off  wind=1  clouds=10  EnableVolumetricClouds=off  CloudCoverage=0  CloudAltitude=6  fog=0  rain=0  RaindropsEffect=off  SnowDensity=0  EnableGeospatial=off  TilesetSource=Earth terrain  UseTrueOrigin=off  OriginHeight=200  OriginLatitude=40.744652  OriginLongitude=-73.988864  MapStyle=Aerial  AdditionalAssetIDs=[]  UseAdvancedSunSky=off  SolarTime=11  TimeZone=-5  Day=21  Month=9  Year=2022  UseDaylightSavingTime=on  DSTStartDay=10  DSTStartMonth=3  DSTEndDay=3  DSTEndMonth=11  DSTSwitchHour=2  sensorTag=MainCamera1  sensorId=1  sensorName=MainCamera1  mountLoc=Origin  offsetFlag=off  tmountOffset=[0, 0, 0]  rmountOffset=[0, 0, 0]  HorizontalResolution=1280  VerticalResolution=720  HorizontalFOV=60  mountPoint=[0 0 0]  mountOrientation=[0 0 0]  aMode=4  ID=1  GeoTrigger=Inactive  ViewNameList={'Custom'}  ViewTranslationList={'[0 0 0]'}  ViewRotationList={'[0 0 0]'}
      settings: LibrarySourceBlock=uavsim3dlib/Simulation 3D Scene Configuration
  Simulation 3D UAV Vehicle : uavsim3dlib/Simulation 3D UAV Vehicle  Priority=-1  Mesh=Quadrotor  MeshPath=/MathWorksUAVContent/UAVs/HexaRotorUAV/HexaRotor.HexaRotor  Color=Silver  ActorName=SimulinkVehicle1  UseGlobalFrame=off  InitialTranslation=[0 0 0]  InitialRotation=[0 0 0]  InitialTranslationGlobal=[0 0 0]  InitialGeoOrigin=[0 0 0]  InitialRotationGlobal=[0 0 0]  SampleTime=0.2  ActorType=SimulinkVehicle  ID=1  aMode=4  ActorTag=SimulinkVehicle1
  Simulation 3D UAV Vehicle1 : uavsim3dlib/Simulation 3D UAV Vehicle  Priority=-1  Mesh=Quadrotor  MeshPath=/MathWorksUAVContent/UAVs/HexaRotorUAV/HexaRotor.HexaRotor  Color=Red  ActorName=SimulinkVehicle2  UseGlobalFrame=off  InitialTranslation=[0 0 0]  InitialRotation=[0 0 0]  InitialTranslationGlobal=[0 0 0]  InitialGeoOrigin=[0 0 0]  InitialRotationGlobal=[0 0 0]  SampleTime=0.2  ActorType=SimulinkVehicle  ID=2  aMode=4  ActorTag=SimulinkVehicle2
  To Multimedia File : dspvision/To Multimedia File  Commented=on  outputFilename=scene.mp4  streamSelection=Video only  videoCompressor=None (uncompressed)  audioCompressor=None (uncompressed)  imagePorts=One multidimensional signal  fileType=MPEG4  audioDatatype=Determine from input data type  fourcc=RGB  audioBitRate=128  audioQuality=75  videoQuality=75  mj2000CompFactor=10
      settings: LibrarySourceBlock=visionsinks/To Multimedia File
  To Video Display : visionsinks/To Video Display  windowSizeMode=Normal  openAtMdlStart=on  fullScreen=off  videoWindowX=536805376  videoWindowY=536805376  saveWindowSize=off  videoWindowWidth=1280  videoWindowHeight=720  inputColorFormat=RGB  inputType=Obsolete  imagePorts=One multidimensional signal  OutputDevice=On-screen video monitor  dataOrg=Column-major  isWindowOpen=off
  wires:
  Gain1/1 -> Simulation 3D UAV Vehicle/2
  Gain/1 -> Simulation 3D UAV Vehicle/1  "NED => Unreal Engine Frame"
  Selector/1 -> Gain1/1
  NED position [m]/1 -> Gain/1
  euler_angles [rad]/1 -> Selector/1
  Constant2/1 -> Selector1/1
  Selector1/1 -> Gain3/1
  Gain2/1 -> Simulation 3D UAV Vehicle1/1
  Gain3/1 -> Simulation 3D UAV Vehicle1/2
  Constant1/1 -> Gain2/1
  Simulation 3D Camera/1 -> To Video Display/1, To Multimedia File/1

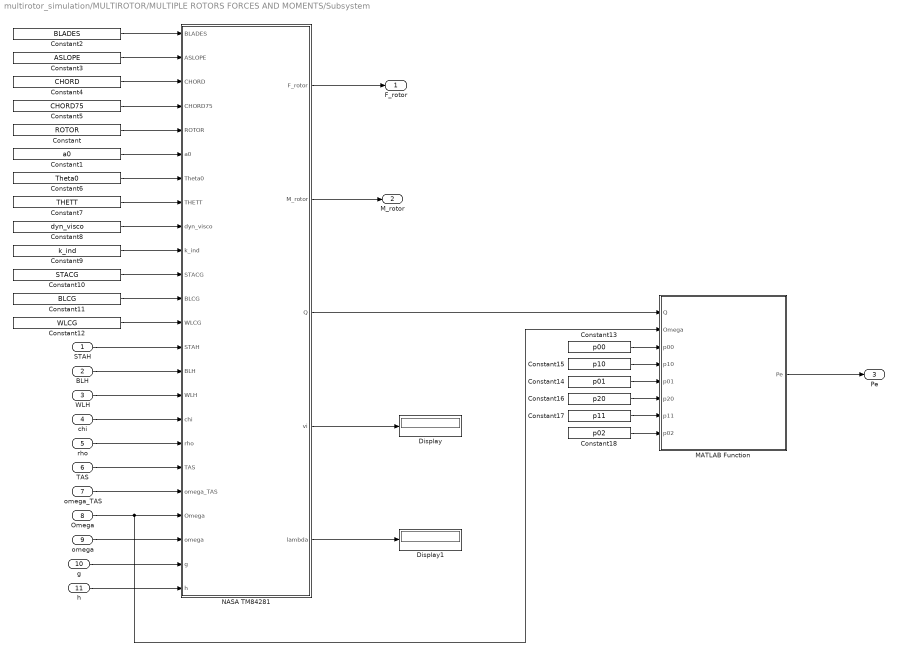
== system multirotor_simulation/MULTIROTOR/MULTIPLE ROTORS FORCES AND MOMENTS/Subsystem ==
  STAH : Inport
  BLH : Inport  Port=2
  WLH : Inport  Port=3
  chi : Inport  Port=4
  rho : Inport  Port=5
  TAS : Inport  Port=6
  omega_TAS : Inport  Port=7
  Omega : Inport  Port=8
  omega : Inport  Port=9
  g : Inport  Port=10
  h : Inport  Port=11
  Constant : Constant  Value=ROTOR
  Constant1 : Constant  Value=a0
  Constant10 : Constant  Value=STACG
  Constant11 : Constant  Value=BLCG
  Constant12 : Constant  Value=WLCG
  Constant13 : Constant  Value=p00
  Constant14 : Constant  Value=p01
  Constant15 : Constant  Value=p10
  Constant16 : Constant  Value=p20
  Constant17 : Constant  Value=p11
  Constant18 : Constant  Value=p02
  Constant2 : Constant  Value=BLADES
  Constant3 : Constant  Value=ASLOPE
  Constant4 : Constant  Value=CHORD
  Constant5 : Constant  Value=CHORD75
  Constant6 : Constant  Value=Theta0
  Constant7 : Constant  Value=THETT
  Constant8 : Constant  Value=dyn_visco
  Constant9 : Constant  Value=k_ind
  Display : Display
  Display1 : Display
  MATLAB Function : MATLAB Function  TreatAsAtomicUnit=on
  NASA TM84281 : MATLAB Function  TreatAsAtomicUnit=on
  F_rotor : Outport
  M_rotor : Outport  Port=2
  Pe : Outport  Port=3
  wires:
  STAH/1 -> NASA TM84281/14(STAH)
  Constant2/1 -> NASA TM84281/1(BLADES)
  Constant1/1 -> NASA TM84281/6(a0)
  Constant17/1 -> MATLAB Function/7(p11)
  NASA TM84281/5(lambda) -> Display1/1
  rho/1 -> NASA TM84281/18(rho)
  omega/1 -> NASA TM84281/22(omega)
  h/1 -> NASA TM84281/24(h)
  Constant/1 -> NASA TM84281/5(ROTOR)
  Constant6/1 -> NASA TM84281/7(Theta0)
  Constant16/1 -> MATLAB Function/6(p20)
  Constant11/1 -> NASA TM84281/12(BLCG)
  Constant3/1 -> NASA TM84281/2(ASLOPE)
  NASA TM84281/1(F_rotor) -> F_rotor/1
  Constant7/1 -> NASA TM84281/8(THETT)
  Constant10/1 -> NASA TM84281/11(STACG)
  BLH/1 -> NASA TM84281/15(BLH)
  Constant4/1 -> NASA TM84281/3(CHORD)
  Constant5/1 -> NASA TM84281/4(CHORD75)
  WLH/1 -> NASA TM84281/16(WLH)
  Omega/1 -> NASA TM84281/21(Omega), MATLAB Function/2(Omega)
  Constant13/1 -> MATLAB Function/3(p00)
  NASA TM84281/3(Q) -> MATLAB Function/1(Q)
  Constant9/1 -> NASA TM84281/10(k_ind)
  NASA TM84281/2(M_rotor) -> M_rotor/1
  Constant8/1 -> NASA TM84281/9(dyn_visco)
  Constant12/1 -> NASA TM84281/13(WLCG)
  NASA TM84281/4(vi) -> Display/1
  TAS/1 -> NASA TM84281/19(TAS)
  MATLAB Function/1(Pe) -> Pe/1
  Constant14/1 -> MATLAB Function/5(p01)
  omega_TAS/1 -> NASA TM84281/20(omega_TAS)
  g/1 -> NASA TM84281/23(g)
  chi/1 -> NASA TM84281/17(chi)
  Constant15/1 -> MATLAB Function/4(p10)
  Constant18/1 -> MATLAB Function/8(p02)

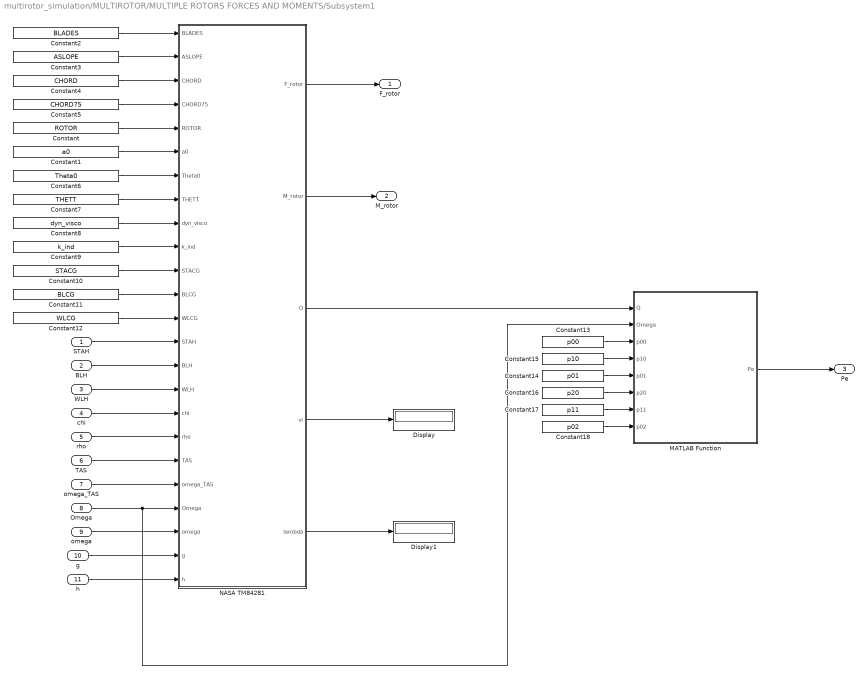
== system multirotor_simulation/MULTIROTOR/MULTIPLE ROTORS FORCES AND MOMENTS/Subsystem1 ==
  STAH : Inport
  BLH : Inport  Port=2
  WLH : Inport  Port=3
  chi : Inport  Port=4
  rho : Inport  Port=5
  TAS : Inport  Port=6
  omega_TAS : Inport  Port=7
  Omega : Inport  Port=8
  omega : Inport  Port=9
  g : Inport  Port=10
  h : Inport  Port=11
  Constant : Constant  Value=ROTOR
  Constant1 : Constant  Value=a0
  Constant10 : Constant  Value=STACG
  Constant11 : Constant  Value=BLCG
  Constant12 : Constant  Value=WLCG
  Constant13 : Constant  Value=p00
  Constant14 : Constant  Value=p01
  Constant15 : Constant  Value=p10
  Constant16 : Constant  Value=p20
  Constant17 : Constant  Value=p11
  Constant18 : Constant  Value=p02
  Constant2 : Constant  Value=BLADES
  Constant3 : Constant  Value=ASLOPE
  Constant4 : Constant  Value=CHORD
  Constant5 : Constant  Value=CHORD75
  Constant6 : Constant  Value=Theta0
  Constant7 : Constant  Value=THETT
  Constant8 : Constant  Value=dyn_visco
  Constant9 : Constant  Value=k_ind
  Display : Display
  Display1 : Display
  MATLAB Function : MATLAB Function  TreatAsAtomicUnit=on
  NASA TM84281 : MATLAB Function  TreatAsAtomicUnit=on
  F_rotor : Outport
  M_rotor : Outport  Port=2
  Pe : Outport  Port=3
  wires:
  STAH/1 -> NASA TM84281/14(STAH)
  Constant2/1 -> NASA TM84281/1(BLADES)
  Constant1/1 -> NASA TM84281/6(a0)
  Constant17/1 -> MATLAB Function/7(p11)
  NASA TM84281/5(lambda) -> Display1/1
  rho/1 -> NASA TM84281/18(rho)
  omega/1 -> NASA TM84281/22(omega)
  h/1 -> NASA TM84281/24(h)
  Constant/1 -> NASA TM84281/5(ROTOR)
  Constant6/1 -> NASA TM84281/7(Theta0)
  Constant16/1 -> MATLAB Function/6(p20)
  Constant11/1 -> NASA TM84281/12(BLCG)
  Constant3/1 -> NASA TM84281/2(ASLOPE)
  NASA TM84281/1(F_rotor) -> F_rotor/1
  Constant7/1 -> NASA TM84281/8(THETT)
  Constant10/1 -> NASA TM84281/11(STACG)
  BLH/1 -> NASA TM84281/15(BLH)
  Constant4/1 -> NASA TM84281/3(CHORD)
  Constant5/1 -> NASA TM84281/4(CHORD75)
  WLH/1 -> NASA TM84281/16(WLH)
  Omega/1 -> NASA TM84281/21(Omega), MATLAB Function/2(Omega)
  Constant13/1 -> MATLAB Function/3(p00)
  NASA TM84281/3(Q) -> MATLAB Function/1(Q)
  Constant9/1 -> NASA TM84281/10(k_ind)
  NASA TM84281/2(M_rotor) -> M_rotor/1
  Constant8/1 -> NASA TM84281/9(dyn_visco)
  Constant12/1 -> NASA TM84281/13(WLCG)
  NASA TM84281/4(vi) -> Display/1
  TAS/1 -> NASA TM84281/19(TAS)
  MATLAB Function/1(Pe) -> Pe/1
  Constant14/1 -> MATLAB Function/5(p01)
  omega_TAS/1 -> NASA TM84281/20(omega_TAS)
  g/1 -> NASA TM84281/23(g)
  chi/1 -> NASA TM84281/17(chi)
  Constant15/1 -> MATLAB Function/4(p10)
  Constant18/1 -> MATLAB Function/8(p02)

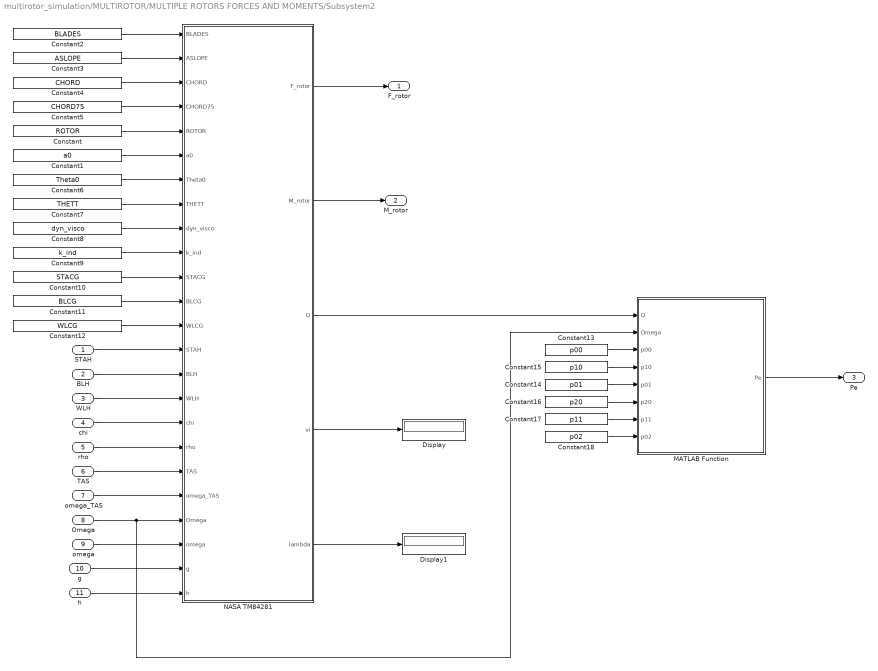
== system multirotor_simulation/MULTIROTOR/MULTIPLE ROTORS FORCES AND MOMENTS/Subsystem2 ==
  STAH : Inport
  BLH : Inport  Port=2
  WLH : Inport  Port=3
  chi : Inport  Port=4
  rho : Inport  Port=5
  TAS : Inport  Port=6
  omega_TAS : Inport  Port=7
  Omega : Inport  Port=8
  omega : Inport  Port=9
  g : Inport  Port=10
  h : Inport  Port=11
  Constant : Constant  Value=ROTOR
  Constant1 : Constant  Value=a0
  Constant10 : Constant  Value=STACG
  Constant11 : Constant  Value=BLCG
  Constant12 : Constant  Value=WLCG
  Constant13 : Constant  Value=p00
  Constant14 : Constant  Value=p01
  Constant15 : Constant  Value=p10
  Constant16 : Constant  Value=p20
  Constant17 : Constant  Value=p11
  Constant18 : Constant  Value=p02
  Constant2 : Constant  Value=BLADES
  Constant3 : Constant  Value=ASLOPE
  Constant4 : Constant  Value=CHORD
  Constant5 : Constant  Value=CHORD75
  Constant6 : Constant  Value=Theta0
  Constant7 : Constant  Value=THETT
  Constant8 : Constant  Value=dyn_visco
  Constant9 : Constant  Value=k_ind
  Display : Display
  Display1 : Display
  MATLAB Function : MATLAB Function  TreatAsAtomicUnit=on
  NASA TM84281 : MATLAB Function  TreatAsAtomicUnit=on
  F_rotor : Outport
  M_rotor : Outport  Port=2
  Pe : Outport  Port=3
  wires:
  STAH/1 -> NASA TM84281/14(STAH)
  Constant2/1 -> NASA TM84281/1(BLADES)
  Constant1/1 -> NASA TM84281/6(a0)
  Constant17/1 -> MATLAB Function/7(p11)
  NASA TM84281/5(lambda) -> Display1/1
  rho/1 -> NASA TM84281/18(rho)
  omega/1 -> NASA TM84281/22(omega)
  h/1 -> NASA TM84281/24(h)
  Constant/1 -> NASA TM84281/5(ROTOR)
  Constant6/1 -> NASA TM84281/7(Theta0)
  Constant16/1 -> MATLAB Function/6(p20)
  Constant11/1 -> NASA TM84281/12(BLCG)
  Constant3/1 -> NASA TM84281/2(ASLOPE)
  NASA TM84281/1(F_rotor) -> F_rotor/1
  Constant7/1 -> NASA TM84281/8(THETT)
  Constant10/1 -> NASA TM84281/11(STACG)
  BLH/1 -> NASA TM84281/15(BLH)
  Constant4/1 -> NASA TM84281/3(CHORD)
  Constant5/1 -> NASA TM84281/4(CHORD75)
  WLH/1 -> NASA TM84281/16(WLH)
  Omega/1 -> NASA TM84281/21(Omega), MATLAB Function/2(Omega)
  Constant13/1 -> MATLAB Function/3(p00)
  NASA TM84281/3(Q) -> MATLAB Function/1(Q)
  Constant9/1 -> NASA TM84281/10(k_ind)
  NASA TM84281/2(M_rotor) -> M_rotor/1
  Constant8/1 -> NASA TM84281/9(dyn_visco)
  Constant12/1 -> NASA TM84281/13(WLCG)
  NASA TM84281/4(vi) -> Display/1
  TAS/1 -> NASA TM84281/19(TAS)
  MATLAB Function/1(Pe) -> Pe/1
  Constant14/1 -> MATLAB Function/5(p01)
  omega_TAS/1 -> NASA TM84281/20(omega_TAS)
  g/1 -> NASA TM84281/23(g)
  chi/1 -> NASA TM84281/17(chi)
  Constant15/1 -> MATLAB Function/4(p10)
  Constant18/1 -> MATLAB Function/8(p02)

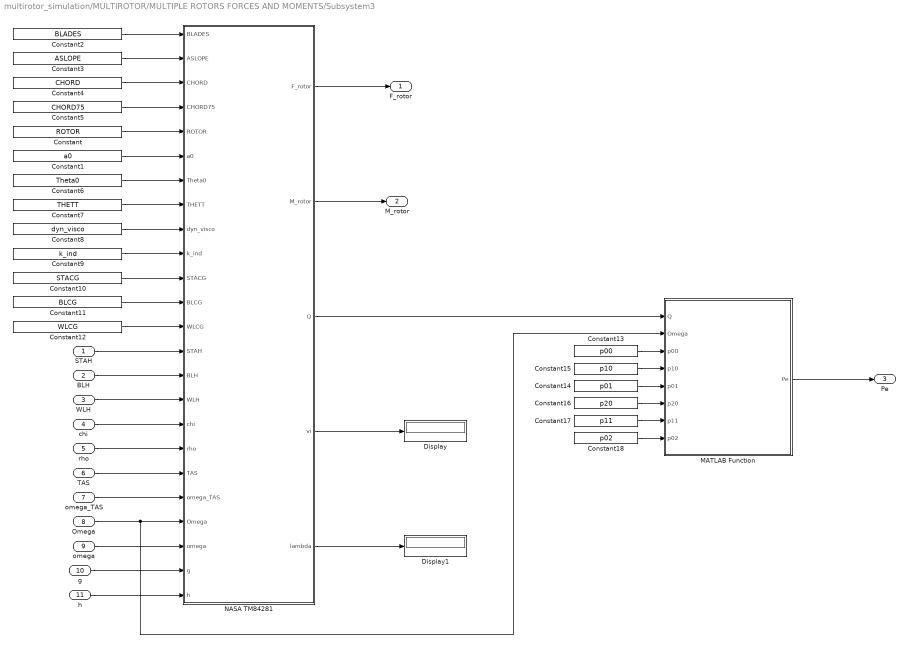
== system multirotor_simulation/MULTIROTOR/MULTIPLE ROTORS FORCES AND MOMENTS/Subsystem3 ==
  STAH : Inport
  BLH : Inport  Port=2
  WLH : Inport  Port=3
  chi : Inport  Port=4
  rho : Inport  Port=5
  TAS : Inport  Port=6
  omega_TAS : Inport  Port=7
  Omega : Inport  Port=8
  omega : Inport  Port=9
  g : Inport  Port=10
  h : Inport  Port=11
  Constant : Constant  Value=ROTOR
  Constant1 : Constant  Value=a0
  Constant10 : Constant  Value=STACG
  Constant11 : Constant  Value=BLCG
  Constant12 : Constant  Value=WLCG
  Constant13 : Constant  Value=p00
  Constant14 : Constant  Value=p01
  Constant15 : Constant  Value=p10
  Constant16 : Constant  Value=p20
  Constant17 : Constant  Value=p11
  Constant18 : Constant  Value=p02
  Constant2 : Constant  Value=BLADES
  Constant3 : Constant  Value=ASLOPE
  Constant4 : Constant  Value=CHORD
  Constant5 : Constant  Value=CHORD75
  Constant6 : Constant  Value=Theta0
  Constant7 : Constant  Value=THETT
  Constant8 : Constant  Value=dyn_visco
  Constant9 : Constant  Value=k_ind
  Display : Display
  Display1 : Display
  MATLAB Function : MATLAB Function  TreatAsAtomicUnit=on
  NASA TM84281 : MATLAB Function  TreatAsAtomicUnit=on
  F_rotor : Outport
  M_rotor : Outport  Port=2
  Pe : Outport  Port=3
  wires:
  STAH/1 -> NASA TM84281/14(STAH)
  Constant2/1 -> NASA TM84281/1(BLADES)
  Constant1/1 -> NASA TM84281/6(a0)
  Constant17/1 -> MATLAB Function/7(p11)
  NASA TM84281/5(lambda) -> Display1/1
  rho/1 -> NASA TM84281/18(rho)
  omega/1 -> NASA TM84281/22(omega)
  h/1 -> NASA TM84281/24(h)
  Constant/1 -> NASA TM84281/5(ROTOR)
  Constant6/1 -> NASA TM84281/7(Theta0)
  Constant16/1 -> MATLAB Function/6(p20)
  Constant11/1 -> NASA TM84281/12(BLCG)
  Constant3/1 -> NASA TM84281/2(ASLOPE)
  NASA TM84281/1(F_rotor) -> F_rotor/1
  Constant7/1 -> NASA TM84281/8(THETT)
  Constant10/1 -> NASA TM84281/11(STACG)
  BLH/1 -> NASA TM84281/15(BLH)
  Constant4/1 -> NASA TM84281/3(CHORD)
  Constant5/1 -> NASA TM84281/4(CHORD75)
  WLH/1 -> NASA TM84281/16(WLH)
  Constant13/1 -> MATLAB Function/3(p00)
  Constant9/1 -> NASA TM84281/10(k_ind)
  NASA TM84281/2(M_rotor) -> M_rotor/1
  Constant8/1 -> NASA TM84281/9(dyn_visco)
  Constant12/1 -> NASA TM84281/13(WLCG)
  NASA TM84281/4(vi) -> Display/1
  TAS/1 -> NASA TM84281/19(TAS)
  MATLAB Function/1(Pe) -> Pe/1
  Constant14/1 -> MATLAB Function/5(p01)
  omega_TAS/1 -> NASA TM84281/20(omega_TAS)
  g/1 -> NASA TM84281/23(g)
  chi/1 -> NASA TM84281/17(chi)
  Constant15/1 -> MATLAB Function/4(p10)
  Constant18/1 -> MATLAB Function/8(p02)
  NASA TM84281/3(Q) -> MATLAB Function/1(Q)
  Omega/1 -> NASA TM84281/21(Omega), MATLAB Function/2(Omega)
